simulink model "lab3_selfmadeModel"  (R2024b)
settings: Solver=ode45  StartTime=0.0  StopTime=10.0  RelTol=1e-3
undefined symbols (not defined in the file): daq, DiscIntNeverNeededParam, drv, gbox, mld, mot, sens, sIn
libraries: simulink x1
settings Model: Creator=pries  LastModifiedBy=pries

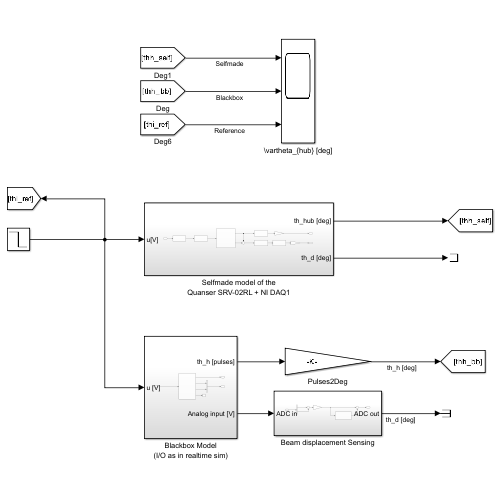
[thumbnail: Simulink's stored preview of the top-level diagram]
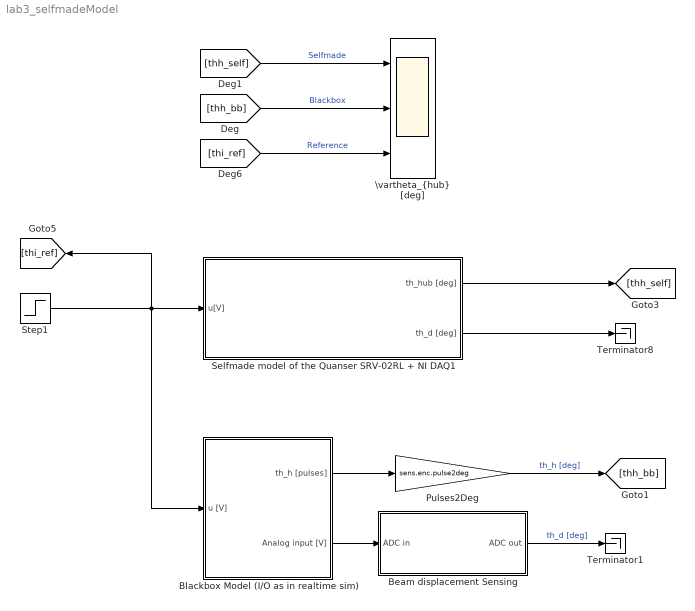
== system lab3_selfmadeModel ==
  Beam displacement Sensing : Subsystem
  Blackbox Model (I/O as in realtime sim) : Subsystem
  Pulses2Deg : Gain  Gain=sens.enc.pulse2deg
  Selfmade model of the Quanser SRV-02RL + NI DAQ1 : Subsystem
  Step1 : Step  Time=0.5  Before=1  After=0  SampleTime=1
  Terminator1 : Terminator
  Terminator8 : Terminator
  "\\vartheta_{hub} [deg]" : Scope  NumInputPorts=3
  wires:
  [thi_ref] -> "\\vartheta_{hub} [deg]"/3  "Reference"
  Step1/1 -> Blackbox Model (I/O as in realtime sim)/1(u [V]), [thi_ref], Selfmade model of the Quanser SRV-02RL + NI DAQ1/1(u[V])
  Selfmade model of the Quanser SRV-02RL + NI DAQ1/2(th_d [deg]) -> Terminator8/1
  [thh_self] -> "\\vartheta_{hub} [deg]"/1  "Selfmade"
  [thh_bb] -> "\\vartheta_{hub} [deg]"/2  "Blackbox"
  Selfmade model of the Quanser SRV-02RL + NI DAQ1/1(th_hub [deg]) -> [thh_self]
  Blackbox Model (I/O as in realtime sim)/2(Analog input [V]) -> Beam displacement Sensing/1(ADC in)
  Blackbox Model (I/O as in realtime sim)/1(th_h [pulses]) -> Pulses2Deg/1
  Beam displacement Sensing/1(ADC out) -> Terminator1/1  "th_d [deg]"
  Pulses2Deg/1 -> [thh_bb]  "th_h [deg]"

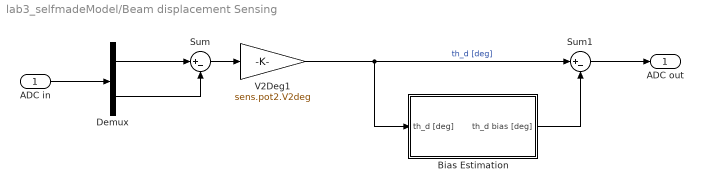
== system lab3_selfmadeModel/Beam displacement Sensing ==
  ADC in : Inport
  Bias Estimation : Subsystem
  Demux : Demux  Outputs=2
  Sum : Sum  Inputs=|+-
  Sum1 : Sum  Inputs=|+-
  V2Deg1 : Gain  Gain=sens.pot2.V2deg
  ADC out : Outport
  wires:
  Bias Estimation/1(th_d bias [deg]) -> Sum1/2
  ADC in/1 -> Demux/1
  V2Deg1/1 -> Bias Estimation/1(th_d [deg]), Sum1/1  "th_d [deg]"
  Sum/1 -> V2Deg1/1
  Demux/2 -> Sum/2
  Demux/1 -> Sum/1
  Sum1/1 -> ADC out/1

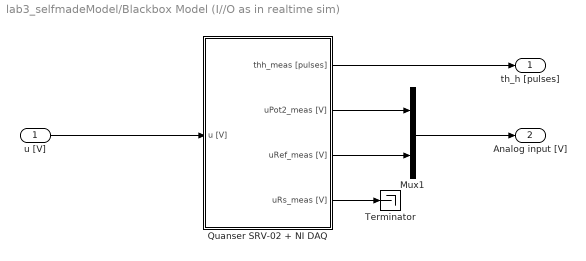
== system lab3_selfmadeModel/Blackbox Model (I//O as in realtime sim) ==
  u [V] : Inport
  Mux1 : Mux  Inputs=2
  Quanser SRV-02 + NI DAQ : Subsystem  mask(Quanser SRV-02 (with resonant load) + NI DAQ){Ts=0.001, fricType=Coulomb + viscous, lockShaft=off, beamInitPos=10}
      mask prompts: Ts "NI DAQ Sample Time:"; fricType "Friction model"; lockShaft "Lock motor shaft"; beamInitPos "Beam initial position [deg]:"
      mask help: Quanser SRV-02 (with resonant load) + NI DAQ model.
      mask init:
      | %%
      | % Riccardo Antonello (riccardo.antonello@unipd.it)
      | %
      | % April 28, 2020
      | %
      | % Dept. of Information Engineering, University of Padova
      | %
      | 
      | %%  Conversion gains
      | deg2rad = pi/180;                   %   [deg]   -> [rad]
      | rad2deg = 180/pi;                   %   [rad]   -> [deg]
      | 
      | 
      | %%  Sensors data
      | 
      | %   shunt resistor
      | sens.curr.Rs = 0.5;   
      | 
      | %   Hewlett-Packard HEDS-5540#A06 optical encoder
      | sens.enc.ppr = 500*4;                                                   %   pulses per rotation
      | sens.enc.pulse2deg = 360/sens.enc.ppr;                                  %   [pulses] -> [deg]
      | sens.enc.pulse2rad = 2*pi/sens.enc.ppr;                                 %   [pulses] -> [rad]
      | sens.enc.deg2pulse = sens.enc.ppr/360;                                  %   [deg] -> [pulses]
      | sens.enc.rad2pulse = sens.enc.ppr/2/pi;                                 %   [rad] -> [pulses]
      | 
      | %   potentiometer 2 (Spectrol 357-0-0-103) - installed on hub
      | sens.pot2.range.R      = 10e3;                                          %   ohmic value range 
      | sens.pot2.range.V      = 5;                                             %   voltage range
      | sens.pot2.range.th_deg = 340;                                           %   angle range [deg]
      | sens.pot2.range.th     = sens.pot2.range.th_deg * deg2rad;              %   angle range [rad]                           
      | sens.pot2.deg2V        = sens.pot2.range.V / sens.pot2.range.th_deg;    %   sensitivity [V/deg]
      | sens.pot2.rad2V        = sens.pot2.range.V / sens.pot2.range.th;        %   sensitivity [V/rad]
      | sens.pot2.V2deg        = 1/sens.pot2.deg2V;                             %   conversion gain [V] -> [deg]
      | sens.pot2.V2rad        = 1/sens.pot2.rad2V;                             %   conversion gain [V] -> [rad]
      | sens.pot2.noise.var    = 3.5e-7;                                        %   out noise variance [V^2]
      | 
      | 
      | %%  Data acquisition board (daq) data
      | 
      | %   NI PCI-6221 DAC data
      | daq.dac.bits = 16;                                  %   resolution (bits)
      | daq.dac.fs   = 10;                                  %   full scale 
      | daq.dac.q    = 2*daq.dac.fs/(2^daq.dac.bits-1);     %	quantization
      | 
      | %   NI PCI-6221 ADC data
      | daq.adc.bits = 16;                                  %   resolution (bits)
      | daq.adc.fs   = 10;                                  %   full scale (as set in SLDRT Analog Input block)
      | daq.adc.q    = 2*daq.adc.fs/(2^daq.adc.bits-1);     %   quantization   
      | 
      | 
      | %%  Set beam initial position
      | % SRV02Handle = find_system(gcb, ...
      | %     'LookUnderMasks', 'on', ...
      | %     'FindAll', 'on', ...
      | %     'FollowLinks', 'on', ...
      | %     'SearchDepth', '1', ...
      | %     'BlockType', 'ModelReference', ...
      | %     'Name', 'Quanser SRV-02');
      | %
      | % %get_param(SRV02Handle, 'InstanceParameters')
      | % InstanceParams = get_param(SRV02Handle, 'InstanceParameters');
      | % for k = 1:length(InstanceParams)
      | %     if strcmp(InstanceParams(k).Name, 'thb0')
      | %         if lockShaft
      | %             InstanceParams(k).Value = sprintf('%f', beamInitPos);
      | %         else
      | %             InstanceParams(k).Value = sprintf('%f', 0);    
      | %         end
      | %         set_param(SRV02Handle, 'InstanceParameters', InstanceParams);
      | %         break;
      | %     end
      | % end
      | 
      | if lockShaft
      |     thb0 = beamInitPos;
      | else
      |     thb0 = 0;    
      | end
      | 
      | 
      | %%  Mask initialization
      | if lockShaft
      |     
      |     %   find Inport handle
      |     InPortHandle = find_system(gcb, ...
      |         'LookUnderMasks', 'on', ...
      |         'FindAll', 'on', ...
      |         'FollowLinks', 'on', ...
      |         'SearchDepth', '1', ...
      |         'BlockType', 'Inport', ...
      |         'Name', 'u [V]');
      |     
      |     if ~isempty(InPortHandle)
      |     
      |         %   find DAC handle
      |         DACHandle = find_system(gcb, ...
      |             'LookUnderMasks', 'on', ...
      |             'FindAll', 'on', ...
      |             'FollowLinks', 'on', ...
      |             'SearchDepth', '1', ...
      |             'BlockType', 'SubSystem', ...
      |             'Name', 'DAC');  
      | 
      |         %   remove Inport output connection   
      |         InportConn = get_param(InPortHandle, 'PortConnectivity');
      |         delete_line(gcb, InportConn.Position);
      | 
      |         %   remove Inport block
      |         delete_block(InPortHandle);
      | 
      |         %   add Constant block
      |         ConstantHandle = add_block( ...
      |             'simulink/Sources/Constant', [gcb, '/u [V]'], ...
      |             'Position', [20   -37    50   -23], ...
      |             'Value', '0');
      | 
      |         %   connect Constant to DAC block
      |         DACPortHandles = get_param(DACHandle, 'PortHandles');
      |         ConstantPortHandles = get_param(ConstantHandle, 'PortHandles');
      |         add_line(gcb, ConstantPortHandles.Outport(1), DACPortHandles.Inport(1));
      |     
      |     end
      |     
      | else
      |     
      |     %   find Constant handle
      |     ConstantHandle = find_system(gcb, ...
      |         'LookUnderMasks', 'on', ...
      |         'FindAll', 'on', ...
      |         'FollowLinks', 'on', ...
      |         'SearchDepth', '1', ...
      |         'BlockType', 'Constant', ...
      |         'Name', 'u [V]');
      |     
      |     if ~isempty(ConstantHandle)
      |     
      |         %   find DAC handle
      |         DACHandle = find_system(gcb, ...
      |             'LookUnderMasks', 'on', ...
      |             'FindAll', 'on', ...
      |             'FollowLinks', 'on', ...
      |             'SearchDepth', '1', ...
      |             'BlockType', 'SubSystem', ...
      |             'Name', 'DAC');  
      |  
      |         %   remove Constant output connection   
      |         ConstantConn = get_param(ConstantHandle, 'PortConnectivity');
      |         delete_line(gcb, ConstantConn.Position);
      | 
      |         %   remove Inport block
      |         delete_block(ConstantHandle);   
      | 
      |         %   add Inport block
      |         InportHandle = add_block( ...
      |             'simulink/Sources/In1', [gcb, '/u [V]'], ...
      |             'Position', [20   -37    50   -23], ...
      |             'Port', '1');
      | 
      |         %   connect Constant to DAC block
      |         DACPortHandles = get_param(DACHandle, 'PortHandles');
      |         InportPortHandles = get_param(InportHandle, 'PortHandles');
      |         add_line(gcb, InportPortHandles.Outport(1), DACPortHandles.Inport(1));
      |     
      |      end
      |     
      | end
      mask Help:
      | Riccardo Antonello (antonello@dei.unipd.it)
      | 
      | April 28, 2020
      | 
      | Dept. of Information Engineering, University of Padova
      mask TypeOptions fricType: Coulomb + viscous | Karnopp
      mask Callback lockShaft:
      | %   get status of check box
      | lockShaft = get_param(gcb, 'lockShaft');
      | 
      | %   get current value of MaskVisibilities property
      | maskVisibilities = get_param(gcb, 'MaskVisibilities');
      | 
      | %   set visibility of the dialog box element
      | if strcmp(lockShaft, 'on')
      |     maskVisibilities{4} = 'on';
      | else
      |     maskVisibilities{4} = 'off';
      | end
      | 
      | % Set the 'MaskVisibilities' property for each parameter in mask
      | set_param( gcb, 'MaskVisibilities', maskVisibilities);
  Terminator : Terminator
  th_h [pulses] : Outport
  Analog input [V] : Outport  Port=2
  wires:
  Quanser SRV-02 + NI DAQ/1(thh_meas [pulses]) -> th_h [pulses]/1
  Quanser SRV-02 + NI DAQ/4(uRs_meas [V]) -> Terminator/1
  Mux1/1 -> Analog input [V]/1
  Quanser SRV-02 + NI DAQ/3(uRef_meas [V]) -> Mux1/2
  Quanser SRV-02 + NI DAQ/2(uPot2_meas [V]) -> Mux1/1
  u [V]/1 -> Quanser SRV-02 + NI DAQ/1(u [V])

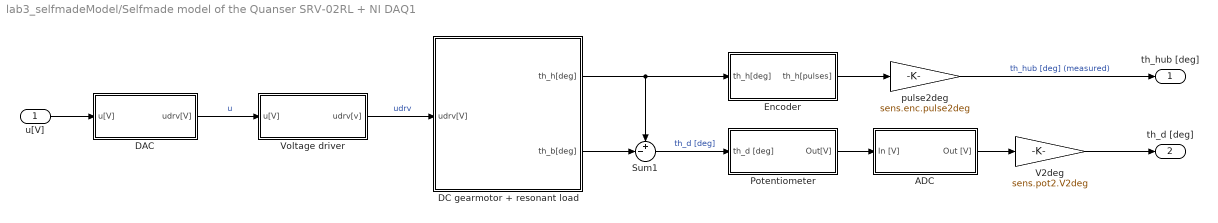
== system lab3_selfmadeModel/Selfmade model of the Quanser SRV-02RL + NI DAQ1 ==
  u[V] : Inport
  ADC : Subsystem
  DAC : Subsystem
  DC gearmotor + resonant load : Subsystem
  Encoder : Subsystem
  Potentiometer : Subsystem
  Sum1 : Sum  Inputs=+-|
  V2deg : Gain  Gain=sens.pot2.V2deg
  Voltage driver : Subsystem
  pulse2deg : Gain  Gain=sens.enc.pulse2deg
  th_hub [deg] : Outport
  th_d [deg] : Outport  Port=2
  wires:
  u[V]/1 -> DAC/1(u[V])
  DAC/1(udrv[V]) -> Voltage driver/1(u[V])  "u"
  Voltage driver/1(udrv[v]) -> DC gearmotor + resonant load/1(udrv[V])  "udrv"
  DC gearmotor + resonant load/1(th_h[deg]) -> Encoder/1(th_h[deg]), Sum1/1
  Encoder/1(th_h[pulses]) -> pulse2deg/1
  pulse2deg/1 -> th_hub [deg]/1  "th_hub [deg] (measured)"
  Potentiometer/1(Out[V]) -> ADC/1(In [V])
  ADC/1(Out [V]) -> V2deg/1
  DC gearmotor + resonant load/2(th_b[deg]) -> Sum1/2
  V2deg/1 -> th_d [deg]/1
  Sum1/1 -> Potentiometer/1(th_d [deg])  "th_d [deg]"

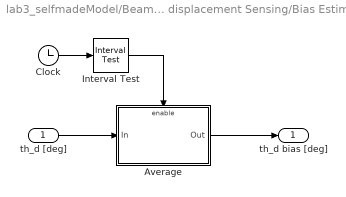
== system lab3_selfmadeModel/Beam displacement Sensing/Bias Estimation ==
  th_d [deg] : Inport
  Average : Subsystem
  Clock : Clock
  Interval Test : simulink/Logic and Bit Operations/Interval Test  IntervalClosedRight=on  uplimit=sIn.t1  IntervalClosedLeft=on  lowlimit=sIn.t0  OutDataTypeStr=boolean
  th_d bias [deg] : Outport
  wires:
  Average/1(Out) -> th_d bias [deg]/1
  th_d [deg]/1 -> Average/1(In)
  Interval Test/1 -> Average/Enable
  Clock/1 -> Interval Test/1

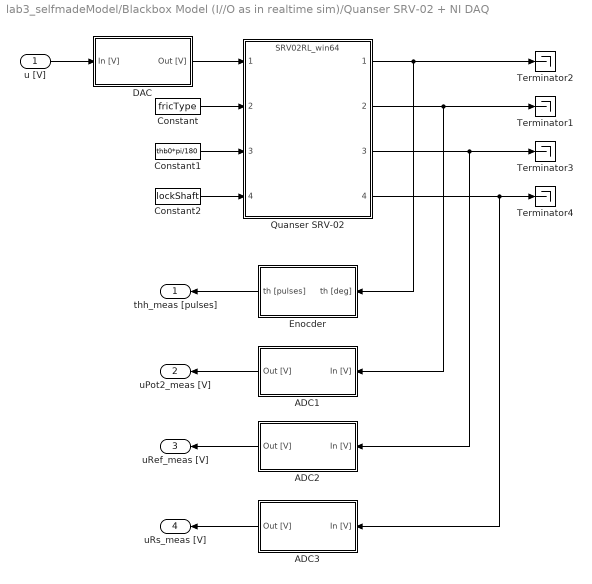
== system lab3_selfmadeModel/Blackbox Model (I//O as in realtime sim)/Quanser SRV-02 + NI DAQ ==
  u [V] : Inport
  ADC1 : Subsystem
  ADC2 : Subsystem
  ADC3 : Subsystem
  Constant : Constant  Value=fricType
  Constant1 : Constant  Value=thb0*pi/180  SampleTime=Inf
  Constant2 : Constant  Value=lockShaft  SampleTime=Inf
  DAC : Subsystem
  Enocder : Subsystem
  Quanser SRV-02 : ModelReference  ModelNameDialog=SRV02RL_win64.slxp  ModelReferenceVersion=1.76  CopyOfModelProtected=on
  Terminator{1..4} (4 alike) : Terminator
  thh_meas [pulses] : Outport
  uPot2_meas [V] : Outport  Port=2
  uRef_meas [V] : Outport  Port=3
  uRs_meas [V] : Outport  Port=4
  wires:
  ADC2/1(Out [V]) -> uRef_meas [V]/1
  Quanser SRV-02/4 -> Terminator4/1, ADC3/1(In [V])
  Constant2/1 -> Quanser SRV-02/4
  Constant1/1 -> Quanser SRV-02/3
  ADC1/1(Out [V]) -> uPot2_meas [V]/1
  Quanser SRV-02/3 -> Terminator3/1, ADC2/1(In [V])
  Constant/1 -> Quanser SRV-02/2
  Quanser SRV-02/1 -> Enocder/1(th [deg]), Terminator2/1
  Quanser SRV-02/2 -> Terminator1/1, ADC1/1(In [V])
  DAC/1(Out [V]) -> Quanser SRV-02/1
  ADC3/1(Out [V]) -> uRs_meas [V]/1
  Enocder/1(th [pulses]) -> thh_meas [pulses]/1
  u [V]/1 -> DAC/1(In [V])

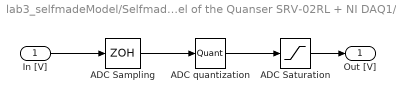
== system lab3_selfmadeModel/Selfmade model of the Quanser SRV-02RL + NI DAQ1/ADC ==
  In [V] : Inport
  ADC Sampling : ZeroOrderHold  SampleTime=daq.adc.Ts
  ADC Saturation : Saturate  UpperLimit=2.5  LowerLimit=-2.5
  ADC quantization : Quantizer  QuantizationInterval=daq.adc.q
  Out [V] : Outport
  wires:
  In [V]/1 -> ADC Sampling/1
  ADC Sampling/1 -> ADC quantization/1
  ADC quantization/1 -> ADC Saturation/1
  ADC Saturation/1 -> Out [V]/1

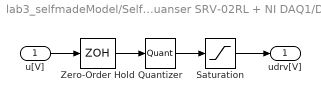
== system lab3_selfmadeModel/Selfmade model of the Quanser SRV-02RL + NI DAQ1/DAC ==
  u[V] : Inport
  Quantizer : Quantizer  QuantizationInterval=daq.dac.q
  Saturation : Saturate  UpperLimit=10  LowerLimit=-10
  Zero-Order Hold : ZeroOrderHold  SampleTime=1e-3
  udrv[V] : Outport
  wires:
  Zero-Order Hold/1 -> Quantizer/1
  u[V]/1 -> Zero-Order Hold/1
  Quantizer/1 -> Saturation/1
  Saturation/1 -> udrv[V]/1

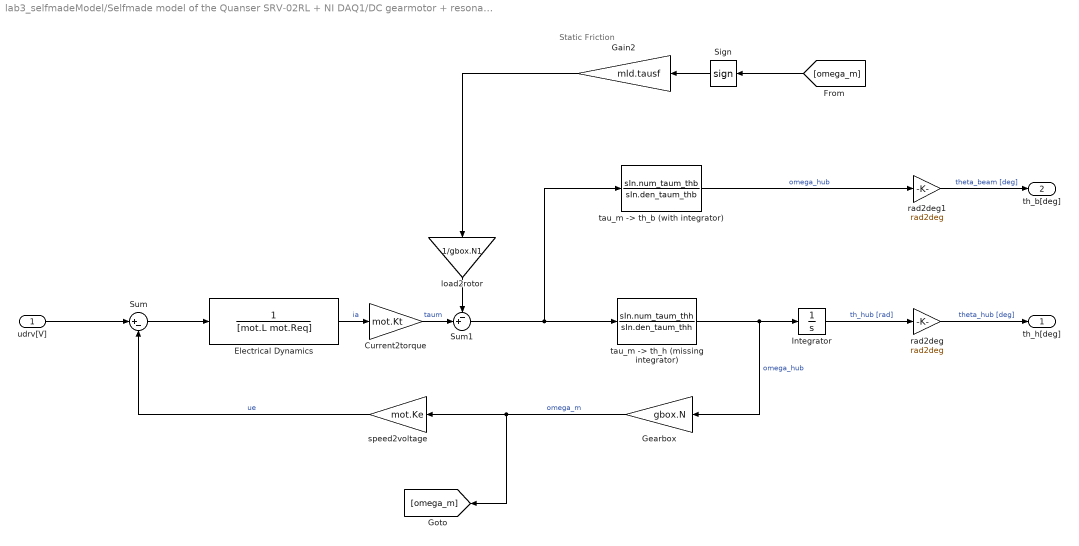
== system lab3_selfmadeModel/Selfmade model of the Quanser SRV-02RL + NI DAQ1/DC gearmotor + resonant load ==
  note: Static Friction
  udrv[V] : Inport
  Current2torque : Gain  Gain=mot.Kt
  Electrical Dynamics : TransferFcn  Denominator=[mot.L mot.Req]
  Gain2 : Gain  Gain=mld.tausf
  Gearbox : Gain  Gain=gbox.N
  Integrator : Integrator
  Sign : Signum  ZeroCross=off
  Sum : Sum  Inputs=|+-
  Sum1 : Sum  Inputs=-+|
  load2rotor : Gain  Gain=1/gbox.N1
  rad2deg : Gain  Gain=rad2deg
  rad2deg1 : Gain  Gain=rad2deg
  speed2voltage : Gain  Gain=mot.Ke
  "tau_m -> th_b (with integrator)" : TransferFcn  Numerator=sIn.num_taum_thb  Denominator=sIn.den_taum_thb
  "tau_m -> th_h (missing integrator)" : TransferFcn  Numerator=sIn.num_taum_thh  Denominator=sIn.den_taum_thh
  th_h[deg] : Outport
  th_b[deg] : Outport  Port=2
  wires:
  rad2deg/1 -> th_h[deg]/1  "theta_hub [deg]"
  [omega_m] -> Sign/1
  Gearbox/1 -> [omega_m], speed2voltage/1  "omega_m"
  load2rotor/1 -> Sum1/1
  speed2voltage/1 -> Sum/2  "ue"
  Electrical Dynamics/1 -> Current2torque/1  "ia"
  Sign/1 -> Gain2/1
  "tau_m -> th_h (missing integrator)"/1 -> Integrator/1, Gearbox/1  "omega_hub"
  Sum1/1 -> "tau_m -> th_b (with integrator)"/1, "tau_m -> th_h (missing integrator)"/1
  Sum/1 -> Electrical Dynamics/1
  Gain2/1 -> load2rotor/1
  Current2torque/1 -> Sum1/2  "taum"
  udrv[V]/1 -> Sum/1
  Integrator/1 -> rad2deg/1  "th_hub [rad]"
  "tau_m -> th_b (with integrator)"/1 -> rad2deg1/1  "omega_hub"
  rad2deg1/1 -> th_b[deg]/1  "theta_beam [deg]"

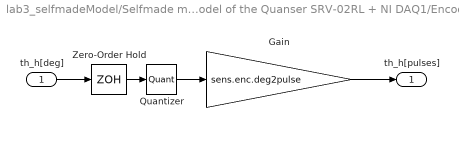
== system lab3_selfmadeModel/Selfmade model of the Quanser SRV-02RL + NI DAQ1/Encoder ==
  th_h[deg] : Inport
  Gain : Gain  Gain=sens.enc.deg2pulse
  Quantizer : Quantizer  QuantizationInterval=sens.enc.pulse2deg
  Zero-Order Hold : ZeroOrderHold  SampleTime=1e-3
  th_h[pulses] : Outport
  wires:
  th_h[deg]/1 -> Zero-Order Hold/1
  Gain/1 -> th_h[pulses]/1
  Quantizer/1 -> Gain/1
  Zero-Order Hold/1 -> Quantizer/1

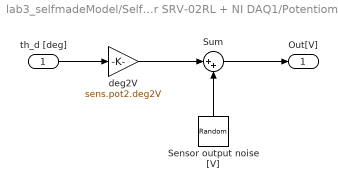
== system lab3_selfmadeModel/Selfmade model of the Quanser SRV-02RL + NI DAQ1/Potentiometer ==
  th_d [deg] : Inport
  Sensor output noise [V] : RandomNumber  Variance=sens.pot2.noise.var  SampleTime=daq.adc.Ts
  Sum : Sum  Inputs=|++
  deg2V : Gain  Gain=sens.pot2.deg2V
  Out[V] : Outport
  wires:
  th_d [deg]/1 -> deg2V/1
  deg2V/1 -> Sum/1
  Sensor output noise [V]/1 -> Sum/2
  Sum/1 -> Out[V]/1

== system lab3_selfmadeModel/Selfmade model of the Quanser SRV-02RL + NI DAQ1/Voltage driver ==
  u[V] : Inport
  Saturation : Saturate  UpperLimit=12  LowerLimit=-12
  Transfer Fcn : TransferFcn  Numerator=[drv.dcgain]  Denominator=[drv.Tc 1]
  udrv[v] : Outport
  wires:
  u[V]/1 -> Transfer Fcn/1
  Transfer Fcn/1 -> Saturation/1
  Saturation/1 -> udrv[v]/1

== system lab3_selfmadeModel/Beam displacement Sensing/Bias Estimation/Average ==
  In : Inport
  Enable : EnablePort
  Discrete-Time Integrator : DiscreteIntegrator  gainval=1/(sIn.t1-sIn.t0)  SampleTime=-1  ICPrevOutput=DiscIntNeverNeededParam  ICPrevScaledInput=DiscIntNeverNeededParam
  Out : Outport
  wires:
  Discrete-Time Integrator/1 -> Out/1
  In/1 -> Discrete-Time Integrator/1

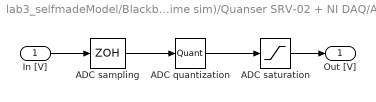
== system lab3_selfmadeModel/Blackbox Model (I//O as in realtime sim)/Quanser SRV-02 + NI DAQ/ADC1 ==
  In [V] : Inport
  ADC quantization : Quantizer  QuantizationInterval=daq.adc.q
  ADC sampling : ZeroOrderHold  SampleTime=Ts
  ADC saturation : Saturate  UpperLimit=daq.adc.fs  LowerLimit=-daq.adc.fs
  Out [V] : Outport
  wires:
  ADC quantization/1 -> ADC saturation/1
  In [V]/1 -> ADC sampling/1
  ADC sampling/1 -> ADC quantization/1
  ADC saturation/1 -> Out [V]/1

== system lab3_selfmadeModel/Blackbox Model (I//O as in realtime sim)/Quanser SRV-02 + NI DAQ/ADC2 ==
  In [V] : Inport
  ADC quantization : Quantizer  QuantizationInterval=daq.adc.q
  ADC sampling : ZeroOrderHold  SampleTime=Ts
  ADC saturation : Saturate  UpperLimit=daq.adc.fs  LowerLimit=-daq.adc.fs
  Out [V] : Outport
  wires:
  ADC saturation/1 -> Out [V]/1
  ADC sampling/1 -> ADC quantization/1
  In [V]/1 -> ADC sampling/1
  ADC quantization/1 -> ADC saturation/1

== system lab3_selfmadeModel/Blackbox Model (I//O as in realtime sim)/Quanser SRV-02 + NI DAQ/ADC3 ==
  In [V] : Inport
  Quantizer : Quantizer  QuantizationInterval=daq.adc.q
  Saturation : Saturate  UpperLimit=daq.adc.fs  LowerLimit=-daq.adc.fs
  Zero-Order Hold : ZeroOrderHold  SampleTime=Ts
  Out [V] : Outport
  wires:
  Zero-Order Hold/1 -> Quantizer/1
  Quantizer/1 -> Saturation/1
  In [V]/1 -> Zero-Order Hold/1
  Saturation/1 -> Out [V]/1

== system lab3_selfmadeModel/Blackbox Model (I//O as in realtime sim)/Quanser SRV-02 + NI DAQ/DAC ==
  In [V] : Inport
  Quantizer : Quantizer  QuantizationInterval=daq.dac.q
  Saturation : Saturate  UpperLimit=daq.dac.fs  LowerLimit=-daq.dac.fs
  Zero-Order Hold : ZeroOrderHold  SampleTime=Ts
  Out [V] : Outport
  wires:
  Saturation/1 -> Out [V]/1
  Zero-Order Hold/1 -> Quantizer/1
  In [V]/1 -> Zero-Order Hold/1
  Quantizer/1 -> Saturation/1

== system lab3_selfmadeModel/Blackbox Model (I//O as in realtime sim)/Quanser SRV-02 + NI DAQ/Enocder ==
  th [deg] : Inport
  Quantizer : Quantizer  QuantizationInterval=sens.enc.pulse2deg
  Zero-Order Hold : ZeroOrderHold  SampleTime=Ts
  deg2pulse : Gain  Gain=sens.enc.deg2pulse
  th [pulses] : Outport
  wires:
  deg2pulse/1 -> th [pulses]/1
  Zero-Order Hold/1 -> Quantizer/1
  th [deg]/1 -> Zero-Order Hold/1
  Quantizer/1 -> deg2pulse/1
